simulink model "Impulse_Para"  (R2013b)
settings: Solver=ode8  StartTime=0  StopTime=50.8  FixedStep=sim_stepSize  MaxStep=0.0001  RelTol=1e-6
undefined symbols (not defined in the file or in its folder): sim_imp, sim_Qgain, sim_zoneVolGain
settings Model: Creator=David  LastModifiedBy=davidveitch
settings SolverCC: NumberNewtonIterations=4
settings DataIOCC: LimitDataPoints=off  SignalLoggingSaveFormat=ModelDataLogs  SaveOutput=off  SignalLogging=off  DSMLogging=off  SaveTime=off  TimeSaveName=d_toutImp
settings OptimizationCC: ExpressionDepthLimit=2147483647
settings DebuggingCC: FcnCallInpInsideContextMsg=EnableAllAsWarning  StateNameClashWarn=warning

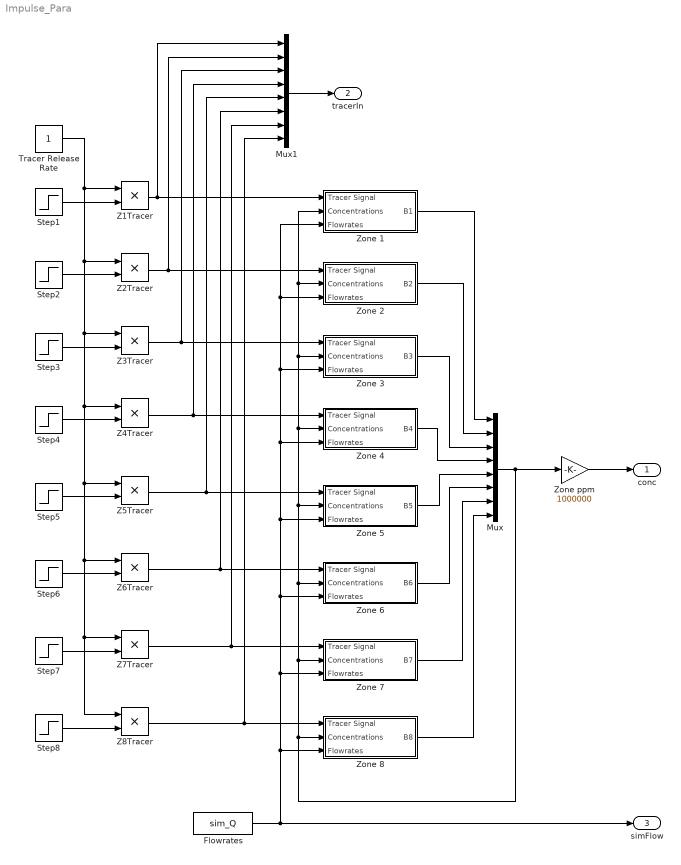
== system Impulse_Para ==
  Flowrates : FromWorkspace  VariableName=sim_Q  SampleTime=0  OutputAfterFinalValue=Holding final value
  Mux : Mux  Inputs=8
  Mux1 : Mux  Inputs=8
  Step1 : Step  Time=1/3600  Before=sim_imp(1)*3600  After=0  SampleTime=0
  Step2 : Step  Time=1/3600  Before=sim_imp(2)*3600  After=0  SampleTime=0
  Step3 : Step  Time=1/3600  Before=sim_imp(3)*3600  After=0  SampleTime=0
  Step4 : Step  Time=1/3600  Before=sim_imp(4)*3600  After=0  SampleTime=0
  Step5 : Step  Time=1/3600  Before=sim_imp(5)*3600  After=0  SampleTime=0
  Step6 : Step  Time=1/3600  Before=sim_imp(6)*3600  After=0  SampleTime=0
  Step7 : Step  Time=1/3600  Before=sim_imp(7)*3600  After=0  SampleTime=0
  Step8 : Step  Time=1/3600  Before=sim_imp(8)*3600  After=0  SampleTime=0
  Tracer Release Rate : Constant
  Z1Tracer : Product  RndMeth=Zero
  Z2Tracer : Product  RndMeth=Zero
  Z3Tracer : Product  RndMeth=Zero
  Z4Tracer : Product  RndMeth=Zero
  Z5Tracer : Product  RndMeth=Zero
  Z6Tracer : Product  RndMeth=Zero
  Z7Tracer : Product  RndMeth=Zero
  Z8Tracer : Product  RndMeth=Zero
  Zone ppm : Gain  Gain=1000000
  Zone 1 : Subsystem
  Zone 2 : Subsystem
  Zone 3 : Subsystem
  Zone 4 : Subsystem
  Zone 5 : Subsystem
  Zone 6 : Subsystem
  Zone 7 : Subsystem
  Zone 8 : Subsystem
  conc : Outport
  tracerIn : Outport  Port=2
  simFlow : Outport  Port=3
  wires:
  Zone 1/1(B1) -> Mux/1
  Zone 2/1(B2) -> Mux/2
  Mux/1 -> Zone ppm/1, Zone 8/2(Concentrations), Zone 7/2(Concentrations), Zone 6/2(Concentrations), Zone 5/2(Concentrations), Zone 4/2(Concentrations), Zone 1/2(Concentrations), Zone 2/2(Concentrations), Zone 3/2(Concentrations)
  Zone 3/1(B3) -> Mux/3
  Z1Tracer/1 -> Mux1/1, Zone 1/1(Tracer Signal)
  Tracer Release Rate/1 -> Z1Tracer/1, Z8Tracer/1, Z7Tracer/1, Z6Tracer/1, Z5Tracer/1, Z4Tracer/1, Z3Tracer/1, Z2Tracer/1
  Z2Tracer/1 -> Zone 2/1(Tracer Signal), Mux1/2
  Z3Tracer/1 -> Zone 3/1(Tracer Signal), Mux1/3
  Flowrates/1 -> simFlow/1, Zone 8/3(Flowrates), Zone 7/3(Flowrates), Zone 6/3(Flowrates), Zone 5/3(Flowrates), Zone 4/3(Flowrates), Zone 3/3(Flowrates), Zone 1/3(Flowrates), Zone 2/3(Flowrates)
  Mux1/1 -> tracerIn/1
  Step1/1 -> Z1Tracer/2
  Step2/1 -> Z2Tracer/2
  Step3/1 -> Z3Tracer/2
  Z4Tracer/1 -> Mux1/4, Zone 4/1(Tracer Signal)
  Step4/1 -> Z4Tracer/2
  Z5Tracer/1 -> Mux1/5, Zone 5/1(Tracer Signal)
  Step5/1 -> Z5Tracer/2
  Zone 4/1(B4) -> Mux/4
  Zone 5/1(B5) -> Mux/5
  Z6Tracer/1 -> Mux1/6, Zone 6/1(Tracer Signal)
  Step6/1 -> Z6Tracer/2
  Z7Tracer/1 -> Mux1/7, Zone 7/1(Tracer Signal)
  Step7/1 -> Z7Tracer/2
  Z8Tracer/1 -> Mux1/8, Zone 8/1(Tracer Signal)
  Step8/1 -> Z8Tracer/2
  Zone 6/1(B6) -> Mux/6
  Zone 7/1(B7) -> Mux/7
  Zone 8/1(B8) -> Mux/8
  Zone ppm/1 -> conc/1

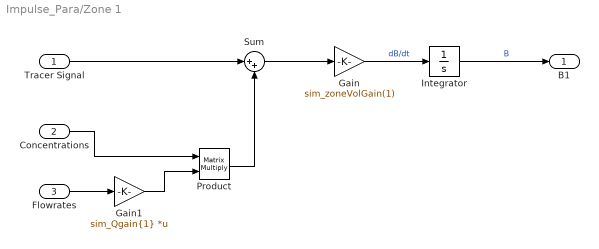
== system Impulse_Para/Zone 1 ==
  Tracer Signal : Inport
  Concentrations : Inport  Port=2
  Flowrates : Inport  Port=3
  Gain : Gain  Gain=sim_zoneVolGain(1)
  Gain1 : Gain  Gain=sim_Qgain{1}  Multiplication=Matrix(K*u)
  Integrator : Integrator
  Product : Product  Multiplication=Matrix(*)  RndMeth=Zero
  Sum : Sum  Inputs=|++
  B1 : Outport
  wires:
  Sum/1 -> Gain/1
  Gain/1 -> Integrator/1  "dB/dt"
  Integrator/1 -> B1/1  "B"
  Concentrations/1 -> Product/1
  Product/1 -> Sum/2
  Tracer Signal/1 -> Sum/1
  Flowrates/1 -> Gain1/1
  Gain1/1 -> Product/2

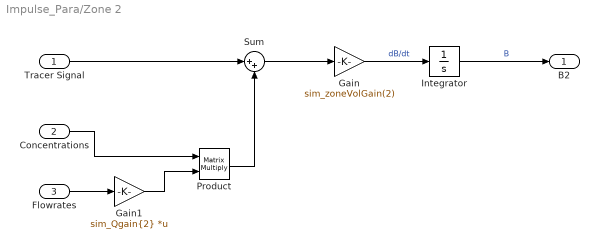
== system Impulse_Para/Zone 2 ==
  Tracer Signal : Inport
  Concentrations : Inport  Port=2
  Flowrates : Inport  Port=3
  Gain : Gain  Gain=sim_zoneVolGain(2)
  Gain1 : Gain  Gain=sim_Qgain{2}  Multiplication=Matrix(K*u)
  Integrator : Integrator
  Product : Product  Multiplication=Matrix(*)  RndMeth=Zero
  Sum : Sum  Inputs=|++
  B2 : Outport
  wires:
  Sum/1 -> Gain/1
  Gain/1 -> Integrator/1  "dB/dt"
  Integrator/1 -> B2/1  "B"
  Concentrations/1 -> Product/1
  Product/1 -> Sum/2
  Tracer Signal/1 -> Sum/1
  Flowrates/1 -> Gain1/1
  Gain1/1 -> Product/2

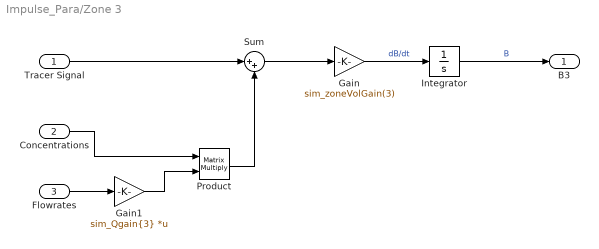
== system Impulse_Para/Zone 3 ==
  Tracer Signal : Inport
  Concentrations : Inport  Port=2
  Flowrates : Inport  Port=3
  Gain : Gain  Gain=sim_zoneVolGain(3)
  Gain1 : Gain  Gain=sim_Qgain{3}  Multiplication=Matrix(K*u)
  Integrator : Integrator
  Product : Product  Multiplication=Matrix(*)  RndMeth=Zero
  Sum : Sum  Inputs=|++
  B3 : Outport
  wires:
  Sum/1 -> Gain/1
  Gain/1 -> Integrator/1  "dB/dt"
  Integrator/1 -> B3/1  "B"
  Concentrations/1 -> Product/1
  Product/1 -> Sum/2
  Tracer Signal/1 -> Sum/1
  Flowrates/1 -> Gain1/1
  Gain1/1 -> Product/2

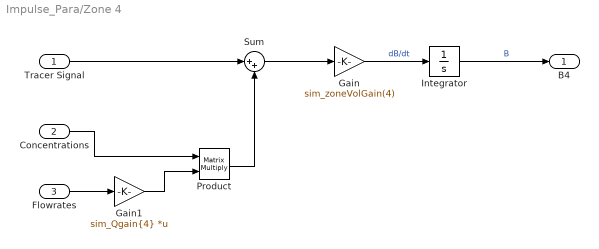
== system Impulse_Para/Zone 4 ==
  Tracer Signal : Inport
  Concentrations : Inport  Port=2
  Flowrates : Inport  Port=3
  Gain : Gain  Gain=sim_zoneVolGain(4)
  Gain1 : Gain  Gain=sim_Qgain{4}  Multiplication=Matrix(K*u)
  Integrator : Integrator
  Product : Product  Multiplication=Matrix(*)  RndMeth=Zero
  Sum : Sum  Inputs=|++
  B4 : Outport
  wires:
  Sum/1 -> Gain/1
  Gain/1 -> Integrator/1  "dB/dt"
  Integrator/1 -> B4/1  "B"
  Concentrations/1 -> Product/1
  Product/1 -> Sum/2
  Tracer Signal/1 -> Sum/1
  Flowrates/1 -> Gain1/1
  Gain1/1 -> Product/2

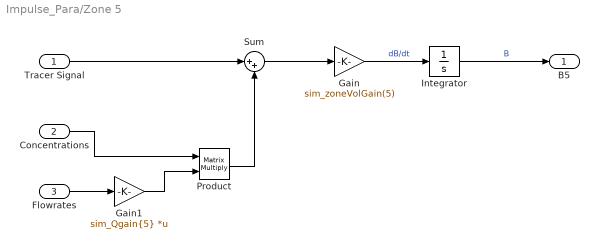
== system Impulse_Para/Zone 5 ==
  Tracer Signal : Inport
  Concentrations : Inport  Port=2
  Flowrates : Inport  Port=3
  Gain : Gain  Gain=sim_zoneVolGain(5)
  Gain1 : Gain  Gain=sim_Qgain{5}  Multiplication=Matrix(K*u)
  Integrator : Integrator
  Product : Product  Multiplication=Matrix(*)  RndMeth=Zero
  Sum : Sum  Inputs=|++
  B5 : Outport
  wires:
  Sum/1 -> Gain/1
  Gain/1 -> Integrator/1  "dB/dt"
  Integrator/1 -> B5/1  "B"
  Concentrations/1 -> Product/1
  Product/1 -> Sum/2
  Tracer Signal/1 -> Sum/1
  Flowrates/1 -> Gain1/1
  Gain1/1 -> Product/2

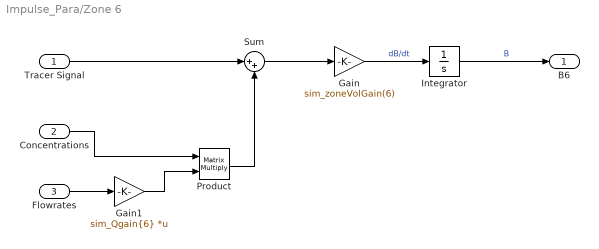
== system Impulse_Para/Zone 6 ==
  Tracer Signal : Inport
  Concentrations : Inport  Port=2
  Flowrates : Inport  Port=3
  Gain : Gain  Gain=sim_zoneVolGain(6)
  Gain1 : Gain  Gain=sim_Qgain{6}  Multiplication=Matrix(K*u)
  Integrator : Integrator
  Product : Product  Multiplication=Matrix(*)  RndMeth=Zero
  Sum : Sum  Inputs=|++
  B6 : Outport
  wires:
  Sum/1 -> Gain/1
  Gain/1 -> Integrator/1  "dB/dt"
  Integrator/1 -> B6/1  "B"
  Concentrations/1 -> Product/1
  Product/1 -> Sum/2
  Tracer Signal/1 -> Sum/1
  Flowrates/1 -> Gain1/1
  Gain1/1 -> Product/2

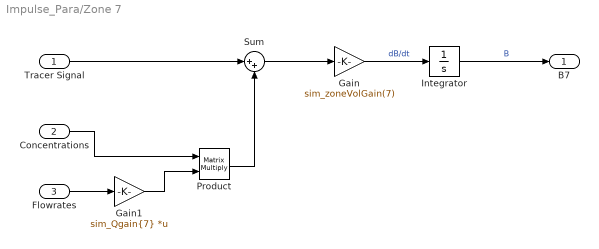
== system Impulse_Para/Zone 7 ==
  Tracer Signal : Inport
  Concentrations : Inport  Port=2
  Flowrates : Inport  Port=3
  Gain : Gain  Gain=sim_zoneVolGain(7)
  Gain1 : Gain  Gain=sim_Qgain{7}  Multiplication=Matrix(K*u)
  Integrator : Integrator
  Product : Product  Multiplication=Matrix(*)  RndMeth=Zero
  Sum : Sum  Inputs=|++
  B7 : Outport
  wires:
  Sum/1 -> Gain/1
  Gain/1 -> Integrator/1  "dB/dt"
  Integrator/1 -> B7/1  "B"
  Concentrations/1 -> Product/1
  Product/1 -> Sum/2
  Tracer Signal/1 -> Sum/1
  Flowrates/1 -> Gain1/1
  Gain1/1 -> Product/2

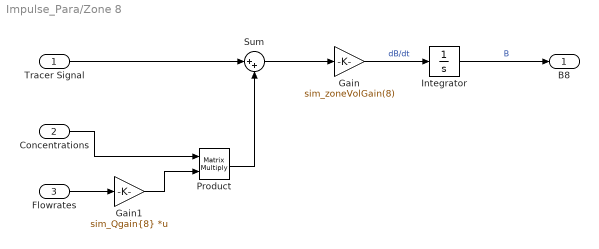
== system Impulse_Para/Zone 8 ==
  Tracer Signal : Inport
  Concentrations : Inport  Port=2
  Flowrates : Inport  Port=3
  Gain : Gain  Gain=sim_zoneVolGain(8)
  Gain1 : Gain  Gain=sim_Qgain{8}  Multiplication=Matrix(K*u)
  Integrator : Integrator
  Product : Product  Multiplication=Matrix(*)  RndMeth=Zero
  Sum : Sum  Inputs=|++
  B8 : Outport
  wires:
  Sum/1 -> Gain/1
  Gain/1 -> Integrator/1  "dB/dt"
  Integrator/1 -> B8/1  "B"
  Concentrations/1 -> Product/1
  Product/1 -> Sum/2
  Tracer Signal/1 -> Sum/1
  Flowrates/1 -> Gain1/1
  Gain1/1 -> Product/2
